simulink model "part_a_model"  (R2020a)
settings: Solver=VariableStepAuto  StartTime=0.0  StopTime=10.0  RelTol=1e-3
libraries: dsparch4 x2
settings Model: Creator=s_moheb  LastModifiedBy=s_moheb

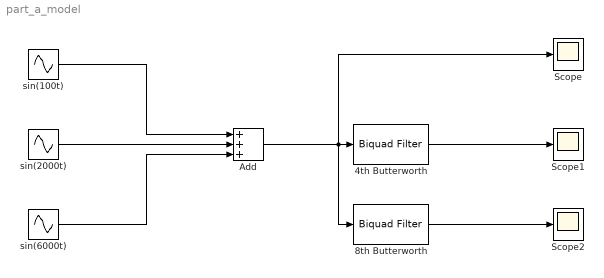
== system part_a_model ==
  4th Butterworth : dsparch4/Biquad Filter  Tag=BlockMethodSubSystem  FilterSource=Dialog parameters  CoeffSource=Specify via dialog  FilterObject=BQF  IIRFiltStruct=Direct form II  BiQuadCoeffs=[1 0 -1 1 0.0540637301548843041 0.945977983156390589;1 0 -1 1 -0.0540637301548842208 0.945977983156392366]  ScaleValues=[0.038214085171932588;0.038214085171932588;1]  IC=0  ICnum=0  ICden=0  a0Flag=Warning  optimizeScaleValues=on  ScaleValueMode=Specify via input port (g)  InputProcessing=Columns as channels (frame based)  roundingMode=Floor  overflowMode=off  scaleValueFracLength=14  denProdOutputFracLength=30  denAccumFracLength=30  secondMemoryFracLength=15
  8th Butterworth : dsparch4/Biquad Filter  Tag=BlockMethodSubSystem  FilterSource=Dialog parameters  CoeffSource=Specify via dialog  FilterObject=BQF  IIRFiltStruct=Direct form II  BiQuadCoeffs=[1 0 -1 1 0.0714856299202889511 0.970412516203148279;1 0 -1 1 -0.071485629920288396 0.9704125162031495;1 0 -1 1 0.0290340881551987562 0.929959622116605433;1 0 -1 1 -0.0290340881551985064 0.929959622116606877]  ScaleValues=[0.0386833765412512715;0.0386833765412512715;0.0379098694572165967;0.0379098694572165967;1]  IC=0  ICnum=0  ICden=0  a0Flag=Warning  optimizeScaleValues=on  ScaleValueMode=Specify via input port (g)  InputProcessing=Columns as channels (frame based)  roundingMode=Floor  overflowMode=off  scaleValueFracLength=14  denProdOutputFracLength=30  denAccumFracLength=30  secondMemoryFracLength=15
  Add : Sum  Inputs=+++
  Scope : Scope
  Scope1 : Scope
  Scope2 : Scope
  sin(100t) : Sin  Frequency=100  SampleTime=1/12000
  sin(2000t) : Sin  Frequency=2000  SampleTime=1/12000
  sin(6000t) : Sin  Frequency=6000  SampleTime=1/12000
  wires:
  sin(100t)/1 -> Add/1
  sin(2000t)/1 -> Add/2
  sin(6000t)/1 -> Add/3
  Add/1 -> 8th Butterworth/1, 4th Butterworth/1, Scope/1
  4th Butterworth/1 -> Scope1/1
  8th Butterworth/1 -> Scope2/1
